simulink model "QuadcopterControlHover"  (R2019b)
settings: Solver=ode4  StartTime=0.0  StopTime=20  FixedStep=1e-3
libraries: simulink x1
settings Model: Creator=bitgar  LastModifiedBy=zczhu

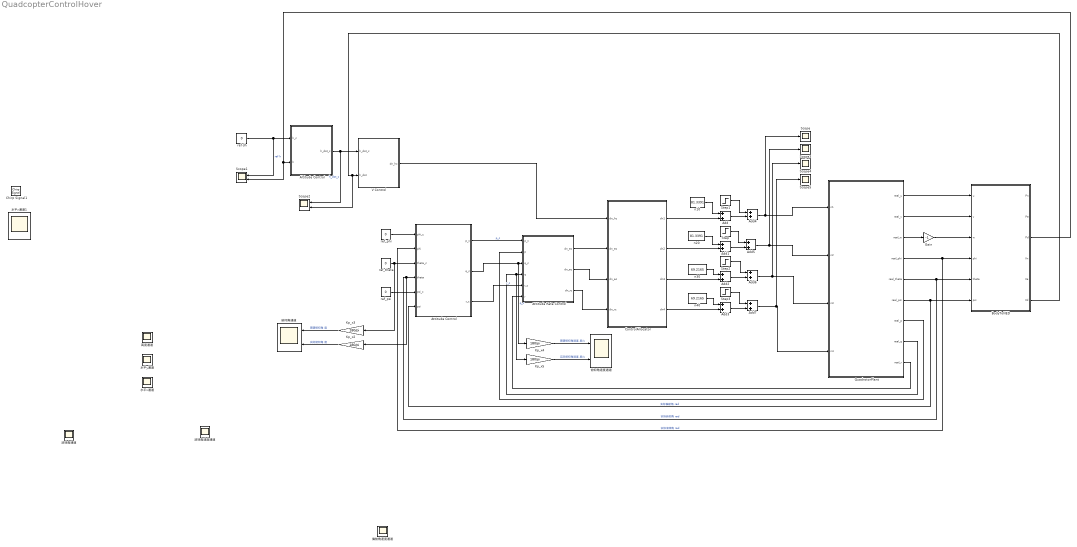
== system QuadcopterControlHover ==
  Add{,1..7} (8 alike) : Sum
  Altitude Control : Subsystem
  Attitude Control : Subsystem
  Attitude Rate Control : Subsystem
  BodyToNED : Subsystem
  Chirp Signal1 : simulink/Sources/Chirp Signal  f1=0.0001  T=100  f2=100
  ControlAllocator : Subsystem
  Gain : Gain  Gain=-1
  Kp_x{2..5} (4 alike) : Gain  Gain=180/pi
  QuadrotorPlant : Subsystem
  Scope{,3..5} (4 alike) : Scope
  Scope1 : Scope  NumInputPorts=2
  Scope2 : Scope  NumInputPorts=2
  Step : Step  Time=10  After=0  SampleTime=0
  Step1 : Step  Time=30  After=0  SampleTime=0
  Step2 : Step  Time=10  After=0  SampleTime=0
  Step3 : Step  Time=10  After=0  SampleTime=0
  V Control : Subsystem
  n10 : Constant  Value=81.3391
  n20 : Constant  Value=81.3391
  n30 : Constant  Value=69.2165
  n40 : Constant  Value=69.2165
  ref dh : Constant  Value=0
  ref_phi : Constant  Value=0
  ref_psi : Constant  Value=0
  ref_theta : Constant  Value=0
  俯仰角通道 : Scope  NumInputPorts=2
  俯仰角速度通道 : Scope  NumInputPorts=2
  偏航角速度通道 : Scope  NumInputPorts=2
  水平x通道 : Scope  NumInputPorts=2
  水平x通道1 : Scope  NumInputPorts=3
  水平y通道 : Scope  NumInputPorts=2
  滚转角通道 : Scope  NumInputPorts=2
  滚转角速度通道 : Scope  NumInputPorts=2
  高度通道 : Scope  NumInputPorts=2
  wires:
  Kp_x2/1 -> 俯仰角通道/2  "实际俯仰角 度"
  Kp_x3/1 -> 俯仰角通道/1  "期望俯仰角 度"
  Kp_x4/1 -> 俯仰角速度通道/1  "期望俯仰角速度 度/s"
  Kp_x5/1 -> 俯仰角速度通道/2  "实际俯仰角速度 度/s"
  QuadrotorPlant/2(real_v) -> BodyToNED/2(v)
  QuadrotorPlant/1(real_u) -> BodyToNED/1(u)
  QuadrotorPlant/3(real_w) -> Gain/1
  QuadrotorPlant/4(real_phi) -> Attitude Control/2(phi), BodyToNED/4(phi)  "实际滚转角 rad"
  QuadrotorPlant/5(real_theta) -> Kp_x2/1, Attitude Control/4(theta), BodyToNED/5(theta)  "实际俯仰角 rad"
  QuadrotorPlant/6(real_psi) -> Attitude Control/6(psi), BodyToNED/6(psi)  "实际偏航角 rad"
  Attitude Control/2(q_c) -> Kp_x4/1, Attitude Rate Control/3(q_c)  "q_c"
  Attitude Control/1(p_c) -> Attitude Rate Control/1(p_c)  "p_c"
  Attitude Control/3(r_c) -> Attitude Rate Control/5(r_c)  "r_c"
  Attitude Rate Control/3(dn_rc) -> ControlAllocator/4(dn_rc)
  Attitude Rate Control/2(dn_ac) -> ControlAllocator/3(dn_ac)
  Attitude Rate Control/1(dn_ec) -> ControlAllocator/2(dn_ec)
  ControlAllocator/1(dn1) -> Add/2
  ControlAllocator/2(dn2) -> Add1/2
  ControlAllocator/3(dn3) -> Add2/2
  ControlAllocator/4(dn4) -> Add3/2
  n10/1 -> Add/1
  n20/1 -> Add1/1
  n30/1 -> Add2/1
  n40/1 -> Add3/1
  Add/1 -> Add4/2
  Add1/1 -> Add5/2
  Add2/1 -> Add6/2
  Add3/1 -> Add7/2
  Step1/1 -> Add4/1
  Step/1 -> Add5/1
  Step2/1 -> Add6/1
  Step3/1 -> Add7/1
  Add4/1 -> Scope/1, QuadrotorPlant/1(n1)
  Add5/1 -> Scope3/1, QuadrotorPlant/2(n2)
  Add6/1 -> Scope4/1, QuadrotorPlant/3(n3)
  Add7/1 -> Scope5/1, QuadrotorPlant/4(n4)
  ref dh/1 -> Scope1/1, Altitude Control/1(h_c)  "ref h"
  Altitude Control/1(h_dot_c) -> Scope2/1, V Control/1(h_dot_c)  "h_dot_c"
  V Control/1(dn_hc) -> ControlAllocator/1(dn_hc)
  QuadrotorPlant/7(real_p) -> Attitude Rate Control/2(p)
  QuadrotorPlant/8(real_q) -> Kp_x5/1, Attitude Rate Control/4(q)
  QuadrotorPlant/9(real_r) -> Attitude Rate Control/6(r)
  ref_phi/1 -> Attitude Control/1(phi_c)
  ref_theta/1 -> Kp_x3/1, Attitude Control/3(theta_c)
  ref_psi/1 -> Attitude Control/5(psi_c)
  BodyToNED/3(Pd) -> Scope1/2, Altitude Control/2(h)
  BodyToNED/6(Vd) -> Scope2/2, V Control/2(h_dot)
  Gain/1 -> BodyToNED/3(w)

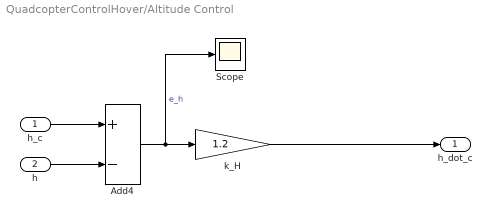
== system QuadcopterControlHover/Altitude Control ==
  h_c : Inport
  h : Inport  Port=2
  Add4 : Sum  Inputs=+-
  Scope : Scope
  k_H : Gain  Gain=1.2
  h_dot_c : Outport
  wires:
  h_c/1 -> Add4/1
  h/1 -> Add4/2
  Add4/1 -> Scope/1, k_H/1  "e_h"
  k_H/1 -> h_dot_c/1

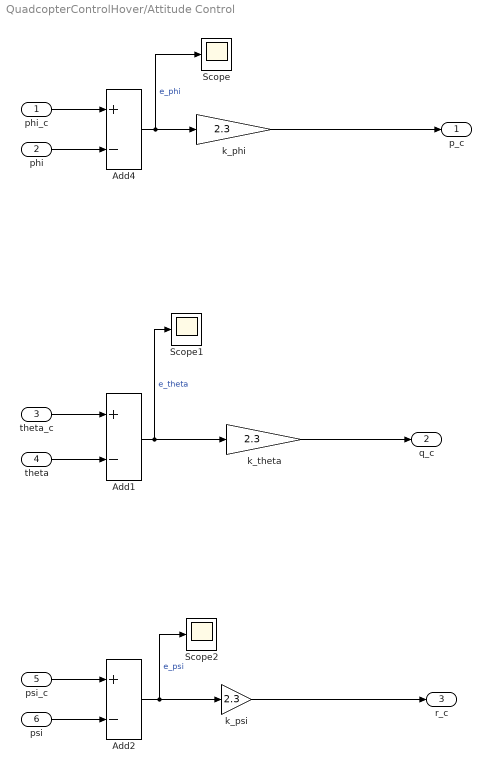
== system QuadcopterControlHover/Attitude Control ==
  phi_c : Inport
  phi : Inport  Port=2
  theta_c : Inport  Port=3
  theta : Inport  Port=4
  psi_c : Inport  Port=5
  psi : Inport  Port=6
  Add1 : Sum  Inputs=+-
  Add2 : Sum  Inputs=+-
  Add4 : Sum  Inputs=+-
  Scope : Scope
  Scope1 : Scope
  Scope2 : Scope
  k_phi : Gain  Gain=2.3
  k_psi : Gain  Gain=2.3
  k_theta : Gain  Gain=2.3
  p_c : Outport
  q_c : Outport  Port=2
  r_c : Outport  Port=3
  wires:
  phi_c/1 -> Add4/1
  phi/1 -> Add4/2
  theta_c/1 -> Add1/1
  theta/1 -> Add1/2
  psi/1 -> Add2/2
  Add4/1 -> Scope/1, k_phi/1  "e_phi"
  psi_c/1 -> Add2/1
  Add1/1 -> Scope1/1, k_theta/1  "e_theta"
  Add2/1 -> Scope2/1, k_psi/1  "e_psi"
  k_phi/1 -> p_c/1
  k_theta/1 -> q_c/1
  k_psi/1 -> r_c/1

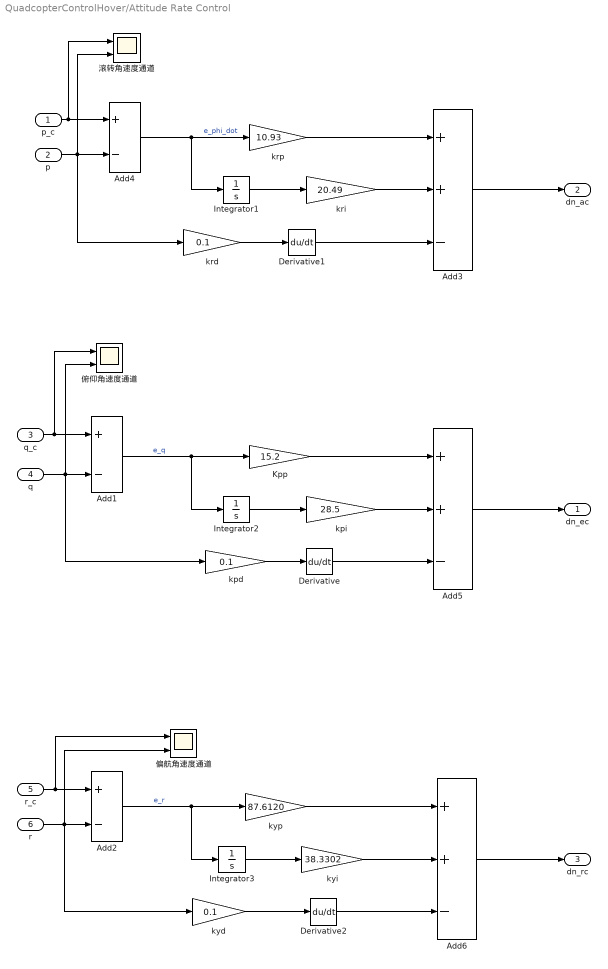
== system QuadcopterControlHover/Attitude Rate Control ==
  p_c : Inport
  p : Inport  Port=2
  q_c : Inport  Port=3
  q : Inport  Port=4
  r_c : Inport  Port=5
  r : Inport  Port=6
  Add1 : Sum  Inputs=+-
  Add2 : Sum  Inputs=+-
  Add3 : Sum  Inputs=++-
  Add4 : Sum  Inputs=+-
  Add5 : Sum  Inputs=++-
  Add6 : Sum  Inputs=++-
  Derivative : Derivative
  Derivative1 : Derivative
  Derivative2 : Derivative
  Integrator1 : Integrator
  Integrator2 : Integrator
  Integrator3 : Integrator
  Kpp : Gain  Gain=15.2
  kpd : Gain  Gain=0.1
  kpi : Gain  Gain=28.5
  krd : Gain  Gain=0.1
  kri : Gain  Gain=20.49
  krp : Gain  Gain=10.93
  kyd : Gain  Gain=0.1
  kyi : Gain  Gain=38.3302
  kyp : Gain  Gain=87.6120
  俯仰角速度通道 : Scope  NumInputPorts=2
  偏航角速度通道 : Scope  NumInputPorts=2
  滚转角速度通道 : Scope  NumInputPorts=2
  dn_ec : Outport
  dn_ac : Outport  Port=2
  dn_rc : Outport  Port=3
  wires:
  p_c/1 -> 滚转角速度通道/1, Add4/1
  p/1 -> krd/1, 滚转角速度通道/2, Add4/2
  q_c/1 -> 俯仰角速度通道/1, Add1/1
  q/1 -> kpd/1, 俯仰角速度通道/2, Add1/2
  r/1 -> 偏航角速度通道/2, kyd/1, Add2/2
  Add4/1 -> Integrator1/1, krp/1  "e_phi_dot"
  r_c/1 -> 偏航角速度通道/1, Add2/1
  Add3/1 -> dn_ac/1
  kri/1 -> Add3/2
  krp/1 -> Add3/1
  Integrator1/1 -> kri/1
  Integrator2/1 -> kpi/1
  Kpp/1 -> Add5/1
  kpi/1 -> Add5/2
  Add1/1 -> Integrator2/1, Kpp/1  "e_q"
  Add5/1 -> dn_ec/1
  Add2/1 -> Integrator3/1, kyp/1  "e_r"
  Integrator3/1 -> kyi/1
  kyp/1 -> Add6/1
  kyi/1 -> Add6/2
  Add6/1 -> dn_rc/1
  kpd/1 -> Derivative/1
  Derivative/1 -> Add5/3
  krd/1 -> Derivative1/1
  Derivative1/1 -> Add3/3
  kyd/1 -> Derivative2/1
  Derivative2/1 -> Add6/3

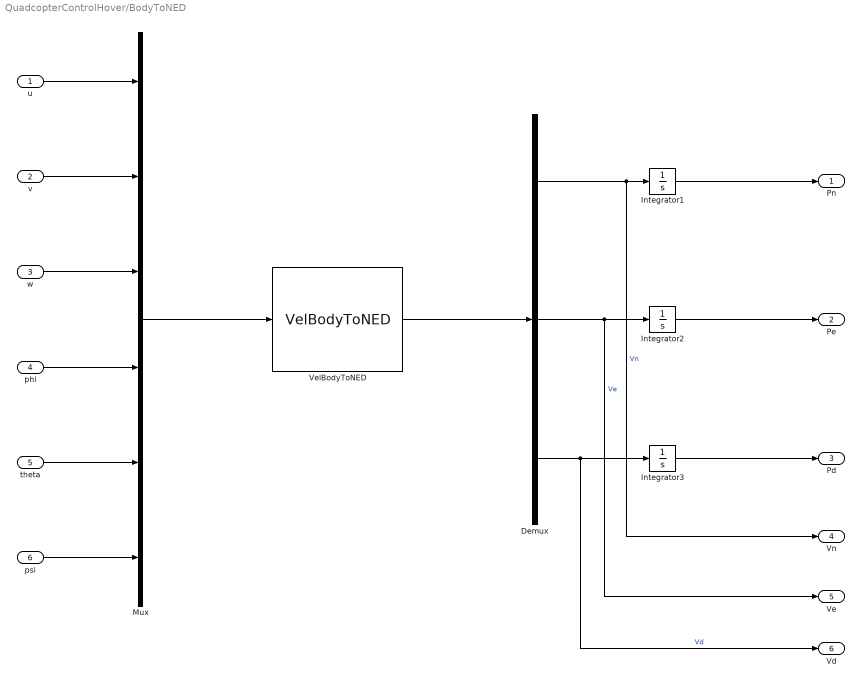
== system QuadcopterControlHover/BodyToNED ==
  u : Inport
  v : Inport  Port=2
  w : Inport  Port=3
  phi : Inport  Port=4
  theta : Inport  Port=5
  psi : Inport  Port=6
  Demux : Demux  Outputs=3
  Integrator1 : Integrator
  Integrator2 : Integrator
  Integrator3 : Integrator
  Mux : Mux  Inputs=6
  VelBodyToNED : S-Function  FunctionName=VelBodyToNED  SFunctionDeploymentMode=off  EnableBusSupport=off
  Pn : Outport
  Pe : Outport  Port=2
  Pd : Outport  Port=3
  Vn : Outport  Port=4
  Ve : Outport  Port=5
  Vd : Outport  Port=6
  wires:
  w/1 -> Mux/3
  psi/1 -> Mux/6
  u/1 -> Mux/1
  v/1 -> Mux/2
  phi/1 -> Mux/4
  theta/1 -> Mux/5
  Mux/1 -> VelBodyToNED/1
  VelBodyToNED/1 -> Demux/1
  Demux/1 -> Vn/1, Integrator1/1  "Vn"
  Demux/3 -> Vd/1, Integrator3/1  "Vd"
  Demux/2 -> Ve/1, Integrator2/1  "Ve"
  Integrator1/1 -> Pn/1
  Integrator3/1 -> Pd/1
  Integrator2/1 -> Pe/1

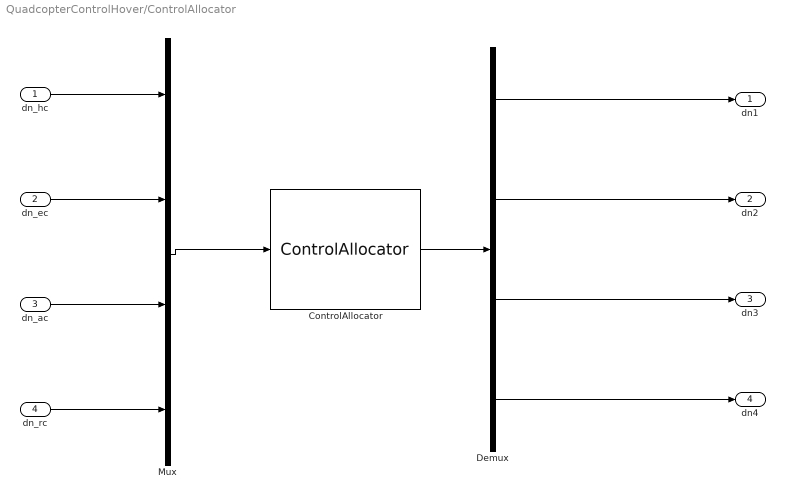
== system QuadcopterControlHover/ControlAllocator ==
  dn_hc : Inport
  dn_ec : Inport  Port=2
  dn_ac : Inport  Port=3
  dn_rc : Inport  Port=4
  ControlAllocator : S-Function  FunctionName=ControlAllocator  Parameters=0.52 0.7107  SFunctionDeploymentMode=off  EnableBusSupport=off
  Demux : Demux
  Mux : Mux
  dn1 : Outport
  dn2 : Outport  Port=2
  dn3 : Outport  Port=3
  dn4 : Outport  Port=4
  wires:
  Demux/2 -> dn2/1
  Demux/1 -> dn1/1
  Demux/3 -> dn3/1
  Demux/4 -> dn4/1
  Mux/1 -> ControlAllocator/1
  dn_ec/1 -> Mux/2
  dn_ac/1 -> Mux/3
  dn_rc/1 -> Mux/4
  ControlAllocator/1 -> Demux/1
  dn_hc/1 -> Mux/1

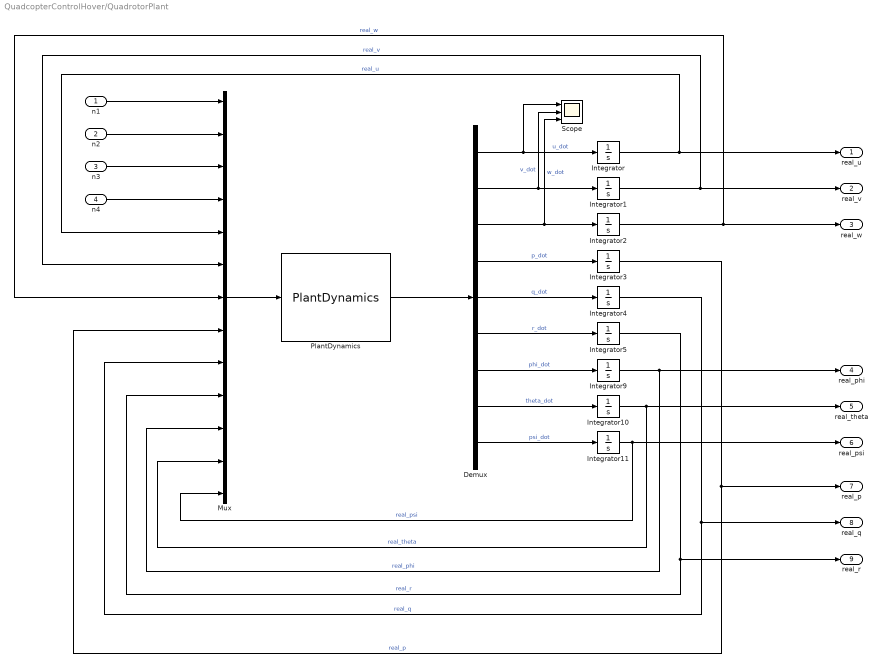
== system QuadcopterControlHover/QuadrotorPlant ==
  n1 : Inport
  n2 : Inport  Port=2
  n3 : Inport  Port=3
  n4 : Inport  Port=4
  Demux : Demux  Outputs=9
  Integrator{,1..5,9..11} (9 alike) : Integrator
  Mux : Mux  Inputs=13
  PlantDynamics : S-Function  FunctionName=PlantDynamics  Parameters=40.37 9.81 0.52 0.7107 1.375 1.126 0.0184 8.1701e-04 13.59 9.052 21.238 0.348  SFunctionDeploymentMode=off  EnableBusSupport=off
  Scope : Scope  NumInputPorts=3
  real_u : Outport
  real_v : Outport  Port=2
  real_w : Outport  Port=3
  real_phi : Outport  Port=4
  real_theta : Outport  Port=5
  real_psi : Outport  Port=6
  real_p : Outport  Port=7
  real_q : Outport  Port=8
  real_r : Outport  Port=9
  wires:
  Demux/4 -> Integrator3/1  "p_dot"
  Mux/1 -> PlantDynamics/1
  Demux/3 -> Scope/3, Integrator2/1  "w_dot"
  n2/1 -> Mux/2
  Demux/1 -> Scope/1, Integrator/1  "u_dot"
  Demux/5 -> Integrator4/1  "q_dot"
  Demux/6 -> Integrator5/1  "r_dot"
  Demux/2 -> Scope/2, Integrator1/1  "v_dot"
  n4/1 -> Mux/4
  n1/1 -> Mux/1
  n3/1 -> Mux/3
  PlantDynamics/1 -> Demux/1
  Integrator9/1 -> Mux/11, real_phi/1  "real_phi"
  Integrator10/1 -> Mux/12, real_theta/1  "real_theta"
  Integrator11/1 -> Mux/13, real_psi/1  "real_psi"
  Integrator/1 -> Mux/5, real_u/1  "real_u"
  Integrator1/1 -> Mux/6, real_v/1  "real_v"
  Integrator2/1 -> Mux/7, real_w/1  "real_w"
  Demux/7 -> Integrator9/1  "phi_dot"
  Demux/8 -> Integrator10/1  "theta_dot"
  Demux/9 -> Integrator11/1  "psi_dot"
  Integrator3/1 -> Mux/8, real_p/1  "real_p"
  Integrator4/1 -> Mux/9, real_q/1  "real_q"
  Integrator5/1 -> Mux/10, real_r/1  "real_r"

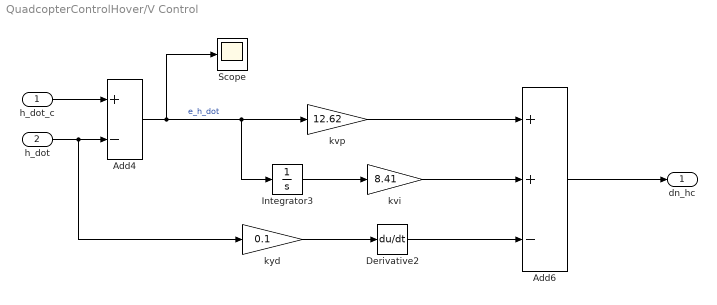
== system QuadcopterControlHover/V Control ==
  h_dot_c : Inport
  h_dot : Inport  Port=2
  Add4 : Sum  Inputs=+-
  Add6 : Sum  Inputs=++-
  Derivative2 : Derivative
  Integrator3 : Integrator
  Scope : Scope
  kvi : Gain  Gain=8.41
  kvp : Gain  Gain=12.62
  kyd : Gain  Gain=0.1
  dn_hc : Outport
  wires:
  h_dot_c/1 -> Add4/1
  h_dot/1 -> kyd/1, Add4/2
  Add4/1 -> Scope/1, Integrator3/1, kvp/1  "e_h_dot"
  Derivative2/1 -> Add6/3
  kyd/1 -> Derivative2/1
  Add6/1 -> dn_hc/1
  kvi/1 -> Add6/2
  Integrator3/1 -> kvi/1
  kvp/1 -> Add6/1
